simulink model "constraints_comparison_A_4D_v2_Fc_connected"  (R2017b)
settings: Solver=ode4  StartTime=0.0  StopTime=total_time  FixedStep=0.001  RelTol=1e-3  EnableMultiTasking=on
InitFcn:
  | % clear
  | % clc
  | 
  | wavelet_gen
undefined symbols (not defined in the file or in its folder): acm_aero_model, acm_T_N, breakpoints1, Cm0, Cmde, Cmq, comp_feedback, constraint_type, dail, de, dele, dele_trim, drud, firstimpulsewidth3211, firstimpulsewidthdoublet, Fr_mp_1, Fr_mp_2, Fr_rp_1, Fr_rp_2, ini_acm_de_deg, ini_acm_p_deg_per_s, ini_acm_phi_deg, ini_acm_psi_deg, ini_acm_q_deg_per_s, ini_acm_r_deg_per_s, ini_acm_theta_deg, ini_cmp_de_deg, ini_rig_p_deg_per_s, ini_rig_phi_deg, ini_rig_psi_deg, ini_rig_q_deg_per_s, ini_rig_r_deg_per_s, ini_rig_theta_deg, input_type, K1_svo_acm, K1_svo_cmp, K2_svo_acm, K2_svo_cmp, La, Ma, max_defl_sat_acm, max_defl_sat_cmp, max_rate_sat, max_rate_sat_acm, max_rate_sat_cmp, Na, radius, sigbuilder_block, simstop, theta_trim, thrust_trim, windspeed, Xa, Ya, Za
libraries: aerolibconvert2 x119, simulink x36, sharedtransform x19, vrlib x2
(part 6 of 6)

== matlab function constraints_comparison_A_4D_v2_Fc_connected/Subsystem14/Subsystem5/MATLAB Function ==
  data: q input; x_ini output; y_ini output; z_ini output
function [x_ini,y_ini,z_ini]= fcn(q)

% Initial position

r = 0.8;

p = [   r
        0
        0   ];

q0 = q(1);
q1 = q(2);
q2 = q(3);
q3 = q(4);

E = [  -q1     q0      -q3     q2
       -q2     q3      q0      -q1
       -q3     -q2     q1      q0  ];
    
E_dash = [     -q1     q0      q3      -q2
               -q2     -q3     q0      q1
               -q3     q2      -q1     q0  ];
           
A = E*transpose(E_dash);

p_in = A*p;

x_ini = p_in(1);
y_ini = p_in(2);
z_ini = p_in(3);

== matlab function constraints_comparison_A_4D_v2_Fc_connected/Subsystem14/Subsystem/MATLAB Function ==
  data: p_rig input; u_ini output; v_ini output; w_ini output; q_rig input; r_rig input; q1 input; q_dot output
function [u_ini,v_ini,w_ini,q_dot]= fcn(p_rig,q_rig,r_rig, q1)

% Initial position
x_ini = -0.38-0.3;
y_ini = 0;
z_ini = 0;

% Local velocities in body axes (Cook, pg.74)
u_ini_body = q_rig*z_ini - r_rig*y_ini;
v_ini_body = r_rig*x_ini - p_rig*z_ini;
w_ini_body = p_rig*y_ini - q_rig*x_ini;

q00 = q1(4);
q11 = q1(5);
q22 = q1(6);
q33 = q1(7);

E = [  -q11     q00      -q33     q22
        -q22     q33      q00      -q11
        -q33     -q22     q11      q00  ];
    
E_dash = [     -q11     q00      q33      -q22
                -q22     -q33     q00      q11
                -q33     q22      -q11     q00  ];

% Body to inertial axes
A = E*transpose(E_dash);

% Inertial axes velocity
V_inertial = A*[    u_ini_body  
                    v_ini_body  
                    w_ini_body      ];
                
u_ini = V_inertial(1);
v_ini = V_inertial(2);
w_ini = V_inertial(3);

q = [   q1(4)
        q1(5)
        q1(6)
        q1(7)    ];

Q = [   -q(2)   -q(3)   -q(4)
        q(1)    -q(4)   q(3)
        q(4)    q(1)    -q(2)
        -q(3)   q(2)    q(1)    ];

omega = [   p_rig
            q_rig
            r_rig       ];

q_dot = 0.5*Q*omega;

== matlab function constraints_comparison_A_4D_v2_Fc_connected/Subsystem14/Subsystem2/MATLAB Function ==
  data: p_rig input; u_ini output; v_ini output; w_ini output; q_rig input; r_rig input; q1 input; q_dot output
function [u_ini,v_ini,w_ini,q_dot]= fcn(p_rig,q_rig,r_rig,q1)

% Initial velocity
% 
% x = 0.129; % 0.2615;
% z = 0.178; % 0.109;
% 
% x_ini = x*cos(theta_rig)+z*sin(theta_rig);
% y_ini = 0;
% z_ini = -x*sin(theta_rig)+z*cos(theta_rig);
% 
% u_ini = q_rig*z_ini; 
% v_ini = 0;
% w_ini = -q_rig*x_ini;

% theta_pos = atan(z/x) - theta_rig;
% r = sqrt(x^2+z^2);
% 
% u_ini = q_rig*r*sin(theta_pos); 
% v_ini = 0;
% w_ini = -q_rig*r*cos(theta_pos);
% 
% q = [   q1(4)
%         q1(5)
%         q1(6)
%         q1(7)    ];
% 
% Q = [   -q(2)   -q(3)   -q(4)
%         q(1)    -q(4)   q(3)
%         q(4)    q(1)    -q(2)
%         -q(3)   q(2)    q(1)    ];
% 
% omega = [   0
%             q_rig
%             0       ];
% 
% q_dot = 0.5*Q*omega;

% Initial position
x_ini = 0.169; % 0.129; % 0.2615;
y_ini = 0;
z_ini = 0.219; % 0.178; % 0.109;

% Local velocities in body axes (Cook, pg.74)
u_ini_body = q_rig*z_ini - r_rig*y_ini;
v_ini_body = r_rig*x_ini - p_rig*z_ini;
w_ini_body = p_rig*y_ini - q_rig*x_ini;

q00 = q1(4);
q11 = q1(5);
q22 = q1(6);
q33 = q1(7);

E = [  -q11     q00      -q33     q22
        -q22     q33      q00      -q11
        -q33     -q22     q11      q00  ];
    
E_dash = [     -q11     q00      q33      -q22
                -q22     -q33     q00      q11
                -q33     q22      -q11     q00  ];

% Body to inertial axes
A = E*transpose(E_dash);

% Inertial axes velocity
V_inertial = A*[    u_ini_body  
                    v_ini_body  
                    w_ini_body      ];
                
u_ini = V_inertial(1);
v_ini = V_inertial(2);
w_ini = V_inertial(3);

q = [   q1(4)
        q1(5)
        q1(6)
        q1(7)    ];

Q = [   -q(2)   -q(3)   -q(4)
        q(1)    -q(4)   q(3)
        q(4)    q(1)    -q(2)
        -q(3)   q(2)    q(1)    ];

omega = [   p_rig
            q_rig
            r_rig       ];

q_dot = 0.5*Q*omega;

== matlab function constraints_comparison_A_4D_v2_Fc_connected/Subsystem14/Subsystem4/MATLAB Function ==
  data: p_rig input; u_ini output; v_ini output; w_ini output; q_rig input; r_rig input; q1 input; qr input; p_acm input; q_dot output; q_acm input; r_acm input
function [u_ini,v_ini,w_ini,q_dot]= fcn(p_rig,q_rig,r_rig,q1,qr,p_acm,q_acm,r_acm)

% Initial position

% r = 0.8;
% 
% x_ini = r*cos(theta_rig);
% y_ini = 0;
% z_ini = -r*sin(theta_rig);
% 
% u_ini = q_rig*z_ini; 
% v_ini = 0;
% w_ini = -q_rig*x_ini;

% Initial position
x_ini = 0.95;
y_ini = 0;
z_ini = 0;

% Local velocities in body axes (Cook, pg.74)
u_ini_body = q_rig*z_ini - r_rig*y_ini;
v_ini_body = r_rig*x_ini - p_rig*z_ini;
w_ini_body = p_rig*y_ini - q_rig*x_ini;

q00 = qr(4);
q11 = qr(5);
q22 = qr(6);
q33 = qr(7);

E = [  -q11     q00      -q33     q22
        -q22     q33      q00      -q11
        -q33     -q22     q11      q00  ];
    
E_dash = [     -q11     q00      q33      -q22
                -q22     -q33     q00      q11
                -q33     q22      -q11     q00  ];

% Body to inertial axes
A = E*transpose(E_dash);

% Inertial axes velocity
V_inertial = A*[    u_ini_body  
                    v_ini_body  
                    w_ini_body      ];
                
u_ini = V_inertial(1);
v_ini = V_inertial(2);
w_ini = V_inertial(3);

q = [   q1(4)
        q1(5)
        q1(6)
        q1(7)    ];

Q = [   -q(2)   -q(3)   -q(4)
        q(1)    -q(4)   q(3)
        q(4)    q(1)    -q(2)
        -q(3)   q(2)    q(1)    ];

omega = [   p_acm
            q_acm
            r_acm       ];

q_dot = 0.5*Q*omega;

== matlab function constraints_comparison_A_4D_v2_Fc_connected/Subsystem14/Extracting aircraft vertical reaction forces1 ==
  data: RF input; RF_a output
function RF_a = fcn(RF)

RF_a = RF(17);

== matlab function constraints_comparison_A_4D_v2_Fc_connected/Subsystem14/Extracting position vector 2/MATLAB Function ==
  data: u input; y output
function y = fcn(u)
%#codegen

y = [   u(1)
        u(2)
        u(3)    ];

== matlab function constraints_comparison_A_4D_v2_Fc_connected/Subsystem14/Extracting position vector 5/MATLAB Function ==
  data: u input; y output
function y = fcn(u)
%#codegen

y = [   u(1)
        u(2)
        u(3)    ];

== matlab function constraints_comparison_A_4D_v2_Fc_connected/Subsystem14/MATLAB Function9 ==
  data: A3 input; A33 output
function A33 = fcn(A3)

A33 = [ A3(1,1)
        A3(2,1)
        A3(3,1)
        A3(1,2)
        A3(2,2)
        A3(3,2)
        A3(1,3)
        A3(2,3)
        A3(3,3) ];

== matlab function constraints_comparison_A_4D_v2_Fc_connected/Subsystem14/MATLAB Function10 ==
  data: A3 input; A33 output
function A33 = fcn(A3)

A33 = [ A3(1,1)
        A3(2,1)
        A3(3,1)
        A3(1,2)
        A3(2,2)
        A3(3,2)
        A3(1,3)
        A3(2,3)
        A3(3,3) ];

== matlab function constraints_comparison_A_4D_v2_Fc_connected/Subsystem14/Subsystem12/MATLAB Function ==
  data: p_rig input; u_ini output; v_ini output; w_ini output; q_rig input; r_rig input; q1 input; q_dot output
function [u_ini,v_ini,w_ini,q_dot]= fcn(p_rig,q_rig,r_rig, q1)

% Initial position

% x = 0.8;
% z = 0.1433;
% 
% theta_pos = atan(z/x) - theta_rig;
% r = sqrt(x^2+z^2);
% 
% u_ini = q_rig*r*sin(theta_pos); 
% v_ini = 0;
% w_ini = -q_rig*r*cos(theta_pos);
% 
% q = [   q1(4)
%         q1(5)
%         q1(6)
%         q1(7)    ];
% 
% Q = [   -q(2)   -q(3)   -q(4)
%         q(1)    -q(4)   q(3)
%         q(4)    q(1)    -q(2)
%         -q(3)   q(2)    q(1)    ];
% 
% omega = [   0
%             q_rig
%             0       ];
% 
% q_dot = 0.5*Q*omega;

% Initial position
x_ini = 0.95;
y_ini = 0;
z_ini = 0.1433;

% Local velocities in body axes (Cook, pg.74)
u_ini_body = q_rig*z_ini - r_rig*y_ini;
v_ini_body = r_rig*x_ini - p_rig*z_ini;
w_ini_body = p_rig*y_ini - q_rig*x_ini;

q00 = q1(4);
q11 = q1(5);
q22 = q1(6);
q33 = q1(7);

E = [  -q11     q00      -q33     q22
        -q22     q33      q00      -q11
        -q33     -q22     q11      q00  ];
    
E_dash = [     -q11     q00      q33      -q22
                -q22     -q33     q00      q11
                -q33     q22      -q11     q00  ];

% Body to inertial axes
A = E*transpose(E_dash);

% Inertial axes velocity
V_inertial = A*[    u_ini_body  
                    v_ini_body  
                    w_ini_body      ];
                
u_ini = V_inertial(1);
v_ini = V_inertial(2);
w_ini = V_inertial(3);

q = [   q1(4)
        q1(5)
        q1(6)
        q1(7)    ];

Q = [   -q(2)   -q(3)   -q(4)
        q(1)    -q(4)   q(3)
        q(4)    q(1)    -q(2)
        -q(3)   q(2)    q(1)    ];

omega = [   p_rig
            q_rig
            r_rig       ];

q_dot = 0.5*Q*omega;

== matlab function constraints_comparison_A_4D_v2_Fc_connected/Subsystem14/Load cell reading to aircraft reaction forces ==
  data: F_acm output; theta_r input; theta_r_dot input; R output size=[3,1]; theta_r_dot_dot input; R_a output; M output; R_reading input; M_reading input; Friction_estimate output
function [F_acm,R,R_a,M,Friction_estimate]= fcn(theta_r,theta_r_dot,theta_r_dot_dot,R_reading,M_reading)

% If a pure tangential force is applied on the aircraft,
% the radial reaction force measured by the load cell is equal to the
% centripetal/centrifugal force created by the aircraft and link.

%% Force to be applied on aircraft in polar coordinates (rig arm axes)
F_acm_r = 10;
F_acm_t = 10;

% Aircraft force to be applied in inertial axes
F_acm_x = +F_acm_r*cos(theta_r)+F_acm_t*sin(theta_r);
F_acm_y = 0;
F_acm_z = -F_acm_r*sin(theta_r)+F_acm_t*cos(theta_r);

F_acm = [   F_acm_x
            F_acm_y
            F_acm_z     ];
        
%% Mass of bodes
m_acm = 1.970;  % kg
m_l = 0.455;    % kg
m_lc = 0.1;     % kg

Iyy_l = 0.00320; % kg.m^2

% Position of body c.g. relative to rig arm gimbal
x_acm = 0.8;    % m
z_acm = 0;      % m
r_acm = sqrt(x_acm^2+z_acm^2);  %m
theta_acm = 0;  % rad

x_l = 0.8;      % m
z_l = 0.1433;	% m
r_l = sqrt(x_l^2+z_l^2);    %m
theta_l = atan(z_l/x_l);	%rad

x_lc = 0.8;     % m
z_lc = 0.3183;	% m
r_lc = sqrt(x_lc^2+z_lc^2);  %m
theta_lc = atan(z_lc/x_lc);	%rad

%% Centrifugal forces of each body (acting radially outward)
F_acm_cent = m_acm*r_acm*theta_r_dot^2;
F_l_cent = m_l*r_l*theta_r_dot^2;
F_lc_cent = m_lc*r_lc*theta_r_dot^2;

% Centrifugal forces in inertial axes
F_acm_cent_x = +F_acm_cent*cos(theta_r);
F_acm_cent_z = -F_acm_cent*sin(theta_r);

F_l_cent_x = +F_l_cent*cos(theta_r-theta_l);
F_l_cent_z = -F_l_cent*sin(theta_r-theta_l);

F_lc_cent_x = +F_lc_cent*cos(theta_r-theta_lc);
F_lc_cent_z = -F_lc_cent*sin(theta_r-theta_lc);

% Total centrifugal force reading on load cell
R_x_cent = F_acm_cent_x + F_l_cent_x;
R_z_cent = F_acm_cent_z + F_l_cent_z;

%% Tangential accelerations of aircraft and link
a_acm_t = -r_acm*theta_r_dot_dot;
a_l_t = -r_l*theta_r_dot_dot;

% Inertial forces from aircraft and link (acting tangentially)
F_acm_in = -m_acm*a_acm_t;
F_l_in = -m_l*a_l_t;

% Inertial forces in inertial axes
F_acm_in_x = F_acm_in*sin(theta_r);
F_acm_in_z = F_acm_in*cos(theta_r);

F_l_in_x = F_l_in*sin(theta_r-theta_l);
F_l_in_z = F_l_in*cos(theta_r-theta_l);

%% Total reaction force reading from load cell [MATCHES TO LOAD CELL REACTION FORCES FROM SIMULATION!]
R = [   R_x_cent + F_acm_in_x + F_l_in_x + F_acm_x
        0
        R_z_cent + F_acm_in_z + F_l_in_z + F_acm_z + (m_acm+m_l)*9.81     ];
    
%% Calculating aircraft reaction force from load cell reading [MATCHES TO AIRCRAFT REACTION FORCES FROM SIMULATION!]
R_a = R_reading - [ F_l_cent_x + F_l_in_x
                    0
                    F_l_cent_z + F_l_in_z + (m_l)*9.81  ];
        
% R_a = R_a*-1;

% Required quantities for calculations:
% Centrifugal forces:       1) Masses and c.g positions of aircraft and link
%                           2) theta_r, theta_r_dot
%
% Inertial force (link):    1) Mass and c.g. postition of link
%                           2) theta_r, theta_r_dot_dot
%
% Weight (link):            1) Mass of link
%
% Summary:  Masses and c.g. positions of aircraft and link
%           theta_r, theta_r_dot, theta_r_dot_dot

%% Load cell moment reading
% All forces * moment arm

% Total forces acting on body c.g. in inertial frame
F_acm_x_total = F_acm_x + F_acm_cent_x + F_acm_in_x;
F_acm_z_total = F_acm_z + F_acm_cent_z + F_acm_in_z + m_acm*9.81;

F_l_x_total = F_l_cent_x + F_l_in_x;
F_l_z_total = F_l_cent_z + F_l_in_z + m_l*9.81;

% Moment contribution for each body on load cell
M_acm = -F_acm_x_total*(z_lc-z_acm)*cos(theta_r) + F_acm_z_total*(z_lc-z_acm)*sin(theta_r);
M_l = -F_l_x_total*(z_lc-z_l)*cos(theta_r) + F_l_z_total*(z_lc-z_l)*sin(theta_r);

M_l_in = -Iyy_l*theta_r_dot_dot; % Additional moment for link (rotational inertial moment)

% Total moment [MATCHES TO PITCHING MOMENT READING FROM SIMULATION!]
M = M_acm + M_l + M_l_in;

% Moment due to aircraft only calculation (need to cancel linear and rotational inertial moments, moment due to weight, and centrifugal moment)
M_acm_from_moment_reading = M_reading - (M_l + M_l_in); % NOTE: difference between this moment and moment calculated using forces will be the friction!
M_acm_from_forces_reading = -R_a(1)*(z_lc-z_acm)*cos(theta_r)+R_a(3)*(z_lc-z_acm)*sin(theta_r);

Friction_estimate = M_acm_from_forces_reading-M_acm_from_moment_reading; % [MATCHES FRICTION INPUT!]

== matlab function constraints_comparison_A_4D_v2_Fc_connected/Subsystem14/Calculating rig pitch acceleration ==
  data: qc input; theta_r_dot_dot output; qc_dot_dot input; theta_r input
function theta_r_dot_dot = fcn(qc,qc_dot_dot,theta_r)

Rc1 = qc(1);
Rc2 = qc(2);
Rc3 = qc(3);
qc0 = qc(4);
qc1 = qc(5);
qc2 = qc(6);
qc3 = qc(7);

Rc1_dot_dot = qc_dot_dot(1);
Rc2_dot_dot = qc_dot_dot(2);
Rc3_dot_dot = qc_dot_dot(3);
qc0_dot_dot = qc_dot_dot(4);
qc1_dot_dot = qc_dot_dot(5);
qc2_dot_dot = qc_dot_dot(6);
qc3_dot_dot = qc_dot_dot(7);

% Transformation matrices
Ec = [  -qc1     qc0      -qc3     qc2
        -qc2     qc3      qc0      -qc1
        -qc3     -qc2     qc1      qc0  ];
    
E_dashc = [     -qc1     qc0      qc3      -qc2
                -qc2     -qc3     qc0      qc1
                -qc3     qc2      -qc1     qc0  ];

Ac = Ec*transpose(E_dashc);


omega_dot_dashc = 2*E_dashc*[	qc0_dot_dot
                                qc1_dot_dot
                                qc2_dot_dot
                                qc3_dot_dot     ];
                            
theta_r_dot_dot = omega_dot_dashc(2);

%% Check using cmp_dot_dot [BOTH METHODS ARE CORRECT]
x_dot_dot = Rc1_dot_dot;
z_dot_dot = Rc3_dot_dot;

t_dot_dot = x_dot_dot*sin(theta_r) + z_dot_dot*cos(theta_r);
    
r = 0.38;
theta_r_dot_dot2 = t_dot_dot/r;

== matlab function constraints_comparison_A_4D_v2_Fc_connected/Subsystem14/Wind axes angular rates calculation ==
  data: qa input size=[7,1]; p output size=[1]; q output size=[1]; qa_wind_dot input size=[4,1]; r output size=[1]; A_b2w output
function [p,q,r,A_b2w] = fcn(qa,qa_wind_dot)

qa0 = qa(4);
qa1 = qa(5);
qa2 = qa(6);
qa3 = qa(7);

qa0_dot = qa_wind_dot(1);
qa1_dot = qa_wind_dot(2);
qa2_dot = qa_wind_dot(3);
qa3_dot = qa_wind_dot(4);

% Transformation matrices
Ea = [  -qa1     qa0      -qa3     qa2
        -qa2     qa3      qa0      -qa1
        -qa3     -qa2     qa1      qa0  ];
    
E_dasha = [     -qa1     qa0      qa3      -qa2
                -qa2     -qa3     qa0      qa1
                -qa3     qa2      -qa1     qa0  ];

A_b2w = Ea*transpose(E_dasha); % body axes to inertial/wind axes transformation

new_E_dasha = Ea;

% Local angular velocities (wind axes)
omega_dasha = 2*E_dasha*[	qa0_dot
                           	qa1_dot
                           	qa2_dot
                           	qa3_dot     ];
                        
% Pitch rate (body axes)
p = omega_dasha(1); % rad/s
q = omega_dasha(2); % rad/s
r = omega_dasha(3); % rad/s

== matlab function constraints_comparison_A_4D_v2_Fc_connected/Subsystem14/HHIRM ==
  data: alpha input size=[1]; beta input size=[1]; p input size=[1]; q input size=[1]; r input size=[1]; dail input; dele input; drud input; A_b2w input; A_b2i input; Fa output; M_dash_a output; CX output; CY output; CZ output; V input
function [Fa,M_dash_a,CX,CY,CZ] = fcn(alpha,beta,p,q,r,dail,dele,drud,A_b2w,A_b2i,V)

rho = 1.225;%1.218; % Density (kg/m^3)

% Reference dimensions (Hawk)
c = 0.143;       % m
S = 0.084942;    % m^2
b = 0.594;       % m

% Reference dimensions (T-tail)
% c = 0.1417;       % m
% S = 0.1077;       % m^2
% b = 0.8967;       % m

ALPHA = alpha;
BETA = beta;
PW_UND=p*b/(2*V);
RW_UND=r*b/(2*V);
QW_UND=q*c/(2*V);

DELTA_e=dele;
DELTA_r=drud;
DELTA_a=dail;
DELTA_dh=0;

DELTA_pp=0;
DELTA_py=0;
DELTA_sp=0;
DELTA_sy=0;
tcs=1.;
tcp=1.;

KCX_tol=0;
KCY_tol=0;
KCZ_tol=0;
KCL_tol=0;
KCM_tol=0;
KCN_tol=0;

%% HHIRM

[CX]=acx(ALPHA,BETA,PW_UND,RW_UND,QW_UND,DELTA_e,...
		DELTA_dh,DELTA_a,DELTA_r,DELTA_pp,DELTA_py,...
		DELTA_sp,DELTA_sy,tcs,tcp,KCX_tol,KCY_tol,...
		KCZ_tol,KCL_tol,KCM_tol,KCN_tol);
    
[CY]=acy(ALPHA,BETA,PW_UND,RW_UND,QW_UND,DELTA_e,...
		DELTA_dh,DELTA_a,DELTA_r,DELTA_pp,DELTA_py,...
		DELTA_sp,DELTA_sy,tcs,tcp,KCX_tol,KCY_tol,...
		KCZ_tol,KCL_tol,KCM_tol,KCN_tol);

[CZ]=acz(ALPHA,BETA,PW_UND,RW_UND,QW_UND,DELTA_e,...
		DELTA_dh,DELTA_a,DELTA_r,DELTA_pp,DELTA_py,...
		DELTA_sp,DELTA_sy,tcs,tcp,KCX_tol,KCY_tol,...
		KCZ_tol,KCL_tol,KCM_tol,KCN_tol);
    
[CL]=acl(ALPHA,BETA,PW_UND,RW_UND,QW_UND,DELTA_e,...
		DELTA_dh,DELTA_a,DELTA_r,DELTA_pp,DELTA_py,...
		DELTA_sp,DELTA_sy,tcs,tcp,KCX_tol,KCY_tol,...
		KCZ_tol,KCL_tol,KCM_tol,KCN_tol);
    
[CM]=acm(ALPHA,BETA,PW_UND,RW_UND,QW_UND,DELTA_e,...
		DELTA_dh,DELTA_a,DELTA_r,DELTA_pp,DELTA_py,...
		DELTA_sp,DELTA_sy,tcs,tcp,KCX_tol,KCY_tol,...
		KCZ_tol,KCL_tol,KCM_tol,KCN_tol);
    
[CN]=acn(ALPHA,BETA,PW_UND,RW_UND,QW_UND,DELTA_e,...
		DELTA_dh,DELTA_a,DELTA_r,DELTA_pp,DELTA_py,...
		DELTA_sp,DELTA_sy,tcs,tcp,KCX_tol,KCY_tol,...
		KCZ_tol,KCL_tol,KCM_tol,KCN_tol);
    
%% Wind axes forces and moments
X=0.5*rho*V^2*S*CX;
Y=0.5*rho*V^2*S*CY;
Z=0.5*rho*V^2*S*CZ;

L=0.5*rho*V^2*S*b*CL;
M=0.5*rho*V^2*S*c*CM;
N=0.5*rho*V^2*S*b*CN;

F_wind = [  X
            Y
            Z   ];
        
M_wind = [  L
            M
            N   ];

%% Body axes forces and moments
F_dash_a = transpose(A_b2w)*F_wind;
M_dash_a = transpose(A_b2w)*M_wind;

%% Inertial axes moments
Fa = A_b2i*F_dash_a;

== matlab function constraints_comparison_A_4D_v2_Fc_connected/Subsystem14/MATLAB Function5 ==
  data: input output; qc input size=[7,1]; qc_dot input size=[7,1]; Vt input; rotation_angles input; s input
function input  = fcn(qc,qc_dot,Vt,rotation_angles,s)
  
Rc1 = qc(1);
Rc2 = qc(2);
Rc3 = qc(3);
qc0 = qc(4);
qc1 = qc(5);
qc2 = qc(6);
qc3 = qc(7);

Rc1_dot = qc_dot(1);
Rc2_dot = qc_dot(2);
Rc3_dot = qc_dot(3);
qc0_dot = qc_dot(4);
qc1_dot = qc_dot(5);
qc2_dot = qc_dot(6);
qc3_dot = qc_dot(7);

% Transformation matrices
Ec = [  -qc1     qc0      -qc3     qc2
        -qc2     qc3      qc0      -qc1
        -qc3     -qc2     qc1      qc0  ];
    
E_dashc = [     -qc1     qc0      qc3      -qc2
                -qc2     -qc3     qc0      qc1
                -qc3     qc2      -qc1     qc0  ];

Ac = Ec*transpose(E_dashc);

% Wind tunnel velocity vector
Vtt = [  Vt
         0   
         0   ];

% Velocity vector of compensator in inertial frame of reference
Vc = [  Rc1_dot
        Rc2_dot
        Rc3_dot	];

% Total velocity vector of compensator in body frame of reference
Vc_dash = transpose(Ac)*(Vc + Vtt);

% Magnitude of total local velocity vector
V0 = sqrt((Vc_dash(1))^2+(Vc_dash(2))^2+(Vc_dash(3))^2);

% Angle of attack
alpha = atan2(Vc_dash(3),Vc_dash(1));

% Sideslip angle [CHECK SIGN]
beta = asin(Vc_dash(2)/V0);

% Local angular velocities
omega_dashc = 2*E_dashc*[	qc0_dot
                            qc1_dot
                            qc2_dot
                            qc3_dot     ];
                        
% Attitude
psi     = rotation_angles(1);
theta   = rotation_angles(2);
phi     = rotation_angles(3);
                        
% Angular rate
p = omega_dashc(1); % rad/s
q = omega_dashc(2); % rad/s
r = omega_dashc(3); % rad/s

x = [   phi
        p
        theta
        q
        psi
        r       ];
    
u = [   s(1)
        s(2)
        s(3)
        s(4)    ];
    
input = [   x
            V0
            u   ];

== matlab function constraints_comparison_A_4D_v2_Fc_connected/Subsystem14/Aircraft loads for load case loop ==
  data: X input; Y input; Fa output size=[3,1]; Z input; L input; M input; N input; M_dash_a output size=[3,1]; A_b2i input
function [Fa,M_dash_a] = fcn(X,Y,Z,L,M,N,A_b2i)

F_dash_a = [    X
                Y
                Z   ];
    
M_dash_a = [    L
                M
                N   ];
            
Fa = A_b2i*F_dash_a;
